simulink model "CrazyPendlm"  (R2014b)
settings: Solver=ode45  StartTime=0.0  StopTime=10  RelTol=1e-3
libraries: vrlib x2
settings Model: Creator=Philipp  LastModifiedBy=sigurd
settings DebuggingCC: UnderspecifiedInitializationDetection=Classic  MergeDetectMultiDrivingBlocksExec=none

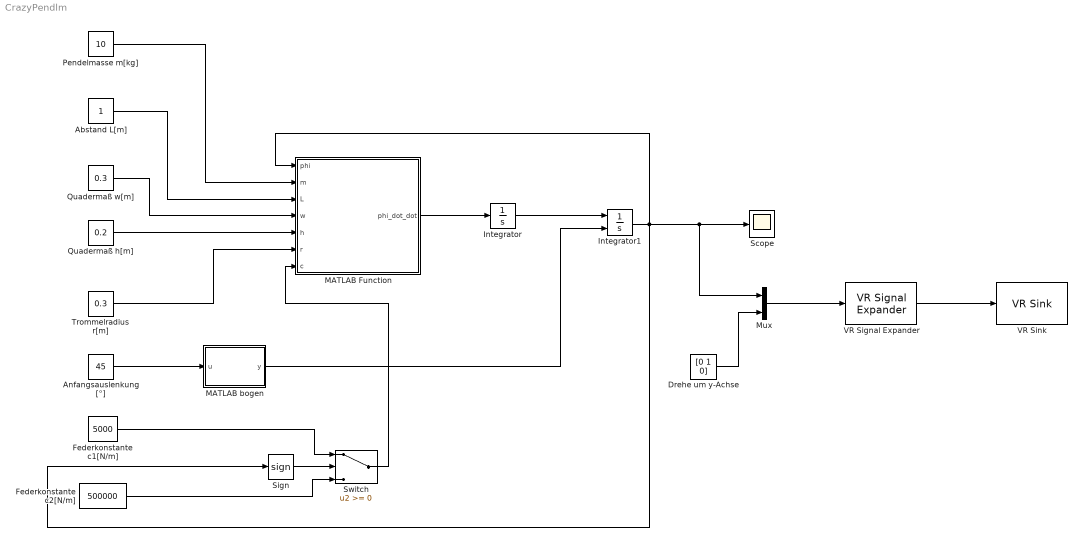
== system CrazyPendlm ==
  Abstand L[m] : Constant
  Anfangsauslenkung [°] : Constant  Value=45
  Drehe um y-Achse : Constant  Value=[0 1 0]
  Federkonstante c1[N/m] : Constant  Value=5000
  Federkonstante c2[N/m] : Constant  Value=500000
  Integrator : Integrator
  Integrator1 : Integrator  InitialConditionSource=external
  MATLAB Function : MATLAB Function  TreatAsAtomicUnit=on
  MATLAB bogen : MATLAB Function  TreatAsAtomicUnit=on
  Mux : Mux  Inputs=2
  Pendelmasse m[kg] : Constant  Value=10
  Quadermaß h[m] : Constant  Value=0.2
  Quadermaß w[m] : Constant  Value=0.3
  Scope : Scope
  Sign : Signum
  Switch : Switch
  Trommelradius r[m] : Constant  Value=0.3
  VR Signal Expander : vrlib/VR Signal Expander  outwidth=4  outidx=[4 1 2 3]
  VR Sink : vrlib/VR Sink  InstantiateOnLoad=on  SampleTime=0.005  ViewEnable=on  RemoteChange=off  RemoteView=off  FieldsWritten=Seiltrommel.rotation.4.1.1.double  WorldFileName=CrazyPendlm.wrl  AutoView=off  VideoDimensions=[]  AllowVariableSize=off
  wires:
  Integrator/1 -> Integrator1/1
  MATLAB Function/1(phi_dot_dot) -> Integrator/1
  MATLAB bogen/1(y) -> Integrator1/2
  Federkonstante c1[N/m]/1 -> Switch/1
  Federkonstante c2[N/m]/1 -> Switch/3
  Integrator1/1 -> Sign/1, MATLAB Function/1(phi), Mux/1, Scope/1
  Pendelmasse m[kg]/1 -> MATLAB Function/2(m)
  Abstand L[m]/1 -> MATLAB Function/3(L)
  Quadermaß w[m]/1 -> MATLAB Function/4(w)
  Quadermaß h[m]/1 -> MATLAB Function/5(h)
  Trommelradius r[m]/1 -> MATLAB Function/6(r)
  Switch/1 -> MATLAB Function/7(c)
  Sign/1 -> Switch/2
  Drehe um y-Achse/1 -> Mux/2
  Mux/1 -> VR Signal Expander/1
  VR Signal Expander/1 -> VR Sink/1
  Anfangsauslenkung [°]/1 -> MATLAB bogen/1(u)

== matlab function CrazyPendlm/MATLAB bogen ==
  data: u input; y output
function y = fcn(u)
%#codegen

y = u*pi/180;

== matlab function CrazyPendlm/MATLAB Function ==
  data: phi input; phi_dot_dot output; m input; L input; w input; h input; r input; c input
function phi_dot_dot = fcn(phi, m, L, w, h, r, c)

g = 9.81;
a = pi/2 - phi;
%a = 90 - phi;

Mg = m * g * sin(phi)*(L+h/2);
Mf = r * r * phi * c;
Js = (1/12 * m * (h^2) + (w^2));
Ja = Js + m * ((L+h/2)*(L+h/2));

phi_dot_dot = ( Mg - Mf ) / ( Ja );
